simulink model "EPA_Jumpe_v1"  (R2018a)
settings: Solver=FixedStepDiscrete  StartTime=0.0  StopTime=inf  FixedStep=0.001  RelTol=1e-3  EnableMultiTasking=on
model workspace (MAT data in the model file):
  k_p_pam = Simulink.Parameter
  k_p_pam.DataType = 'auto'
  k_p_pam.Dimensions = [0 0]
values from neighbouring files (symbols this model uses):
  bits_current = 12    [Init_EPA_Jumper.m]
  bits_GRF = 12    [Init_EPA_Jumper.m]
  bits_Kd = 12    [Init_EPA_Jumper.m]
  bits_Kp = 12    [Init_EPA_Jumper.m]
  bits_position = 16    [Init_EPA_Jumper.m]
  bits_velocity = 12    [Init_EPA_Jumper.m]
  deadzone_in_TIB = 0.45    [Init_EPA_Jumper.m]
  deadzone_out_TIB = 0.48    [Init_EPA_Jumper.m]
  GRF_MAX = 3.3    [Init_EPA_Jumper.m]
  GRF_MIN = 0    [Init_EPA_Jumper.m]
  k_p_TIB = 1    [Init_EPA_Jumper.m]
  KD_MAX = 5.0    (= 5)    [Init_EPA_Jumper.m]
  KD_MIN = 0.0    (= 0)    [Init_EPA_Jumper.m]
  KP_MAX = 500.0    (= 500)    [Init_EPA_Jumper.m]
  KP_MIN = 0.0    (= 0)    [Init_EPA_Jumper.m]
  P_MAX = 95.5    [Init_EPA_Jumper.m]
  P_MIN = -95.5    [Init_EPA_Jumper.m]
  PressureFilter_CutOffFreq = 50    [Init_EPA_Jumper.m]
  PressureFilter_Gain = 1    [Init_EPA_Jumper.m]
  ReadingVoltage = 5    [Init_EPA_Jumper.m]
  T_MAX = 18.0    (= 18)    [Init_EPA_Jumper.m]
  T_MIN = -18.0    (= -18)    [Init_EPA_Jumper.m]
  V_MAX = 45.0    (= 45)    [Init_EPA_Jumper.m]
  V_MIN = -45.0    (= -45)    [Init_EPA_Jumper.m]
  voltageBias_GAS = -2.3721    [Init_EPA_Jumper.m]
  voltageBias_GL = -2.2892    [Init_EPA_Jumper.m]
  voltageBias_HAM = -2.3721    [Init_EPA_Jumper.m]
  voltageBias_IL = -2.3721    [Init_EPA_Jumper.m]
  voltageBias_POP = -2.3721    [Init_EPA_Jumper.m]
  voltageBias_RF = -2.3721    [Init_EPA_Jumper.m]
  voltageBias_SOL = -2.3721    [Init_EPA_Jumper.m]
  voltageBias_TIB = -2.3721    [Init_EPA_Jumper.m]
  voltageBias_VAS = -2.3721    [Init_EPA_Jumper.m]
  voltageMultiplier_GAS = 2.4915    [Init_EPA_Jumper.m]
  voltageMultiplier_GL = 2.5259    [Init_EPA_Jumper.m]
  voltageMultiplier_HAM = 2.4915    [Init_EPA_Jumper.m]
  voltageMultiplier_IL = 2.4915    [Init_EPA_Jumper.m]
  voltageMultiplier_POP = 2.4915    [Init_EPA_Jumper.m]
  voltageMultiplier_RF = 2.4915    [Init_EPA_Jumper.m]
  voltageMultiplier_SOL = 2.4915    [Init_EPA_Jumper.m]
  voltageMultiplier_TIB = 2.4915    [Init_EPA_Jumper.m]
  voltageMultiplier_VAS = 2.4915    [Init_EPA_Jumper.m]
  VoltageResolution = 1024.0    (= 1024)    [Init_EPA_Jumper.m]
libraries: xpcethercatlib x75, simulink x10, peGeneralControl x9, slrtlib x9
(part 1 of 3)
settings Model: xpc_rtwmakecfg_data=_xpcethercatlib_  SimulationMode=external  Creator=marcm  LastModifiedBy=marcm
settings SolverCC: ConcurrentTasks=on  AutoInsertRateTranBlk=on
settings DataIOCC: SaveFormat=StructureWithTime
settings OptimizationCC: BlockReduction=off  OptimizeBlockIOStorage=off  BufferReuse=off  GlobalBufferReuse=off  ExpressionFolding=off  LocalBlockOutputs=off  OptimizeDataStoreBuffers=off  BusAssignmentInplaceUpdate=off
settings HardwareCC: ProdBitPerPointer=32  ProdBitPerSizeT=32  ProdBitPerPtrDiffT=32  ProdLargestAtomicFloat=None  ProdWordSize=32  ProdLongLongMode=on  ProdHWDeviceType=Generic->32-bit x86 compatible
settings RTWCC: SystemTargetFile=slrt.tlc  TemplateMakefile=slrt_default_tmf  Description=Simulink Real-Time  CodeExecutionProfiling=on  RTWCompilerOptimization=on
settings CodeAppCC: StateflowObjectComments=on
settings SimulinkRealTimeCC: SupportVariableSizeSignals=on  xPCConcurrentTasks=on

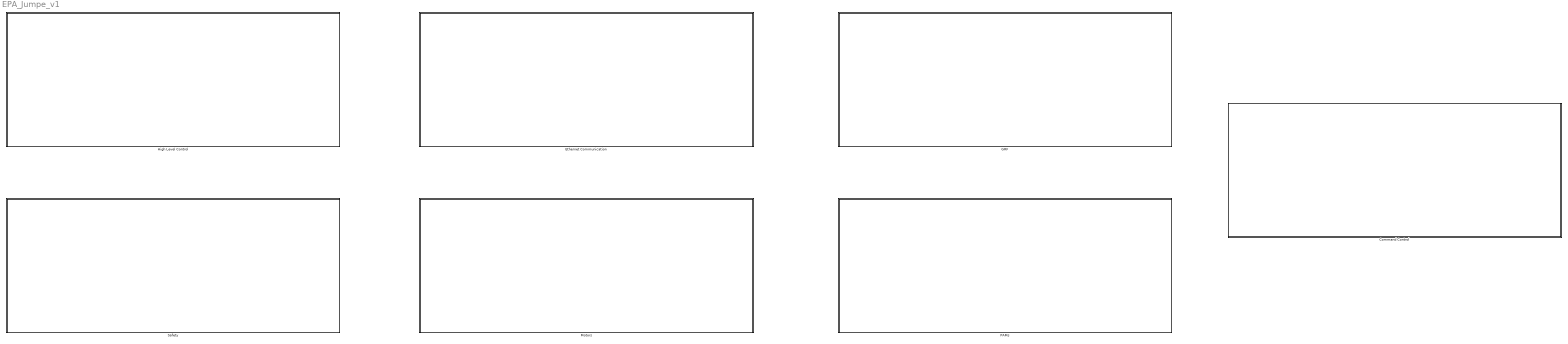
== system EPA_Jumpe_v1 ==
  Command Control : Subsystem
  Ethernet Communication : Subsystem
  GRF : Subsystem
  High Level Control : Subsystem
  Motors : Subsystem
  PAMs : Subsystem
  "Safety " : Subsystem

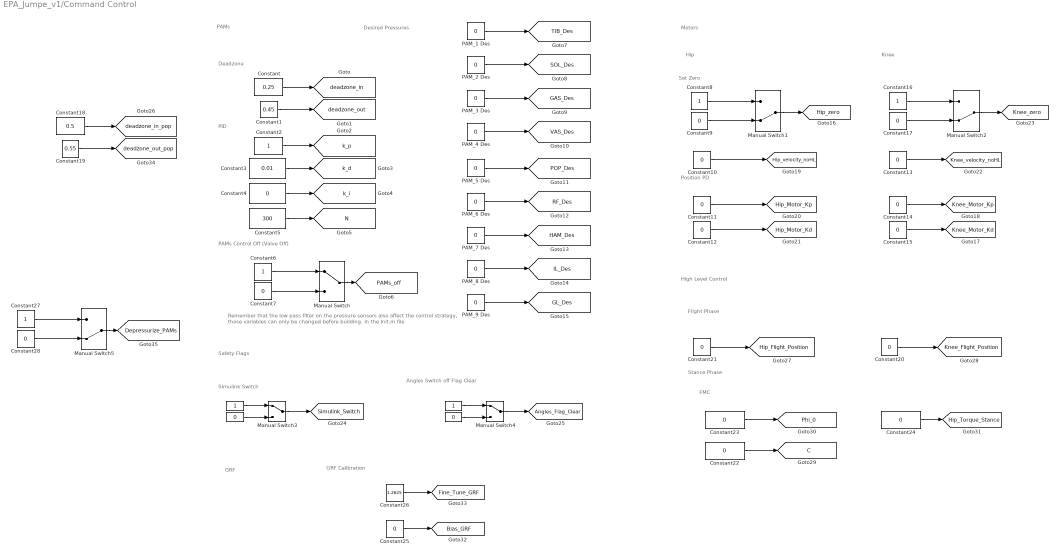
== system EPA_Jumpe_v1/Command Control ==
  note: PID
  note: PAMs
  note: Deadzone
  note: PAMs Control Off (Valve Off)
  note: Desired Pressures
  note: Motors
  note: Remember that the low pass filter on the pressure sensors also affect the control strategy, those variables can only be changed before building. In the Init.m file
  note: Hip
  note: Knee
  note: Safety Flags
  note: Simulink Switch
  note: Angles Switch off Flag Clear
  note: GRF
  note: High Level Control
  note: Flight Phase
  note: Stance Phase
  note: FMC
  note: Position PD
  note: Set Zero
  note: GRF Calibration
  " " : Constant
  "   " : Constant  Value=0
  "    " : Constant  Value=0
  "               " : Constant
  Constant : Constant  Value=0.25
  Constant1 : Constant  Value=0.45
  Constant{4,7,9..15,17,20..25,28} (17 alike) : Constant  Value=0
  Constant{2,6,8,16,27} (5 alike) : Constant
  Constant18 : Constant  Value=0.5
  Constant19 : Constant  Value=0.55
  Constant26 : Constant  Value=1.2625
  Constant3 : Constant  Value=0.01
  Constant5 : Constant  Value=300
  Manual Switch : ManualSwitch
  Manual Switch1 : ManualSwitch  CurrentSetting=0
  Manual Switch2 : ManualSwitch  CurrentSetting=0
  Manual Switch3 : ManualSwitch
  Manual Switch4 : ManualSwitch
  Manual Switch5 : ManualSwitch  CurrentSetting=0
  PAM_1 Des : Constant  Value=0
  PAM_2 Des : Constant  Value=0
  PAM_3 Des : Constant  Value=0
  PAM_4 Des : Constant  Value=0
  PAM_5 Des : Constant  Value=0
  PAM_6 Des : Constant  Value=0
  PAM_7 Des : Constant  Value=0
  PAM_8 Des : Constant  Value=0
  PAM_9 Des : Constant  Value=0
  tag scope: Angles_Flag_Clear=global, Bias_GRF=global, C=global, Depressurize_PAMs=global, Fine_Tune_GRF=global, GAS_Des=global, GL_Des=global, HAM_Des=global, Hip_Flight_Position=global, Hip_Motor_Kd=global, Hip_Motor_Kp=global, Hip_Torque_Stance=global, Hip_velocity_noHL=global, Hip_zero=global, IL_Des=global, Knee_Flight_Position=global, Knee_Motor_Kd=global, Knee_Motor_Kp=global, Knee_velocity_noHL=global, Knee_zero=global, N=global, PAMs_off=global, POP_Des=global, Phi_0=global, RF_Des=global, SOL_Des=global, Simulink_Switch=global, TIB_Des=global, VAS_Des=global, deadzone_in=global, deadzone_in_pop=global, deadzone_out=global, deadzone_out_pop=global, k_d=global, k_i=global, k_p=global
  wires:
  Constant5/1 -> [N]
  Constant4/1 -> [k_i]
  Constant6/1 -> Manual Switch/1
  Manual Switch/1 -> [PAMs_off]
  Constant1/1 -> [deadzone_out]
  Constant7/1 -> Manual Switch/2
  Constant2/1 -> [k_p]
  Constant/1 -> [deadzone_in]
  Constant3/1 -> [k_d]
  PAM_1 Des/1 -> [TIB_Des]
  PAM_2 Des/1 -> [SOL_Des]
  PAM_3 Des/1 -> [GAS_Des]
  PAM_4 Des/1 -> [VAS_Des]
  PAM_5 Des/1 -> [POP_Des]
  PAM_6 Des/1 -> [RF_Des]
  PAM_7 Des/1 -> [HAM_Des]
  PAM_8 Des/1 -> [IL_Des]
  PAM_9 Des/1 -> [GL_Des]
  Constant8/1 -> Manual Switch1/1
  Constant9/1 -> Manual Switch1/2
  Manual Switch1/1 -> [Hip_zero]
  Constant10/1 -> [Hip_velocity_noHL]
  Constant11/1 -> [Hip_Motor_Kp]
  Constant12/1 -> [Hip_Motor_Kd]
  Constant13/1 -> [Knee_velocity_noHL]
  Constant14/1 -> [Knee_Motor_Kp]
  Constant15/1 -> [Knee_Motor_Kd]
  Manual Switch2/1 -> [Knee_zero]
  Constant17/1 -> Manual Switch2/2
  Constant16/1 -> Manual Switch2/1
  " "/1 -> Manual Switch3/1
  "    "/1 -> Manual Switch3/2
  Manual Switch3/1 -> [Simulink_Switch]
  Manual Switch4/1 -> [Angles_Flag_Clear]
  "               "/1 -> Manual Switch4/1
  "   "/1 -> Manual Switch4/2
  Constant21/1 -> [Hip_Flight_Position]
  Constant20/1 -> [Knee_Flight_Position]
  Constant23/1 -> [Phi_0]
  Constant22/1 -> [C]
  Constant24/1 -> [Hip_Torque_Stance]
  Constant25/1 -> [Bias_GRF]
  Constant26/1 -> [Fine_Tune_GRF]
  Constant18/1 -> [deadzone_in_pop]
  Constant19/1 -> [deadzone_out_pop]
  Constant27/1 -> Manual Switch5/1
  Constant28/1 -> Manual Switch5/2
  Manual Switch5/1 -> [Depressurize_PAMs]

== system EPA_Jumpe_v1/Ethernet Communication ==
  "EtherCAT Get Notifications " : xpcethercatlib/EtherCAT Get Notifications   device_id=0  sample_time=.001
      settings: SourceProductName=Simulink Real-Time  SourceProductBaseCode=XP
  "EtherCAT Init " : xpcethercatlib/EtherCAT Init   Priority=0  config_file=C:\Users\marcm\PhD\EPA-Jumper\RealTime Code\EPA Jumper v1\EPA_Jumper_xml.xml  device_id=0  pci_bus=3  pci_slot=0  pci_function=0  dctuning=0  enaDebug=off  enaDC=on  errLink=off  masterDbg=off  stateChgDbg=off  baseClock=off  masterCfg=off  logFile='c:\dbglog.txt'  sample_time=0.001000  DCMode=0
      settings: SourceProductName=Simulink Real-Time  SourceProductBaseCode=XP
  Inputs : Subsystem
  Outputs : Subsystem
  Terminator : Terminator
  Terminator1 : Terminator
  wires:
  "EtherCAT Get Notifications "/1 -> Terminator1/1
  "EtherCAT Init "/1 -> Terminator/1

== system EPA_Jumpe_v1/GRF ==
  note: GRF Meassures
  2D-Vector : Subsystem
  GRFx : Subsystem
  GRFy : Subsystem
  GRFz : Subsystem

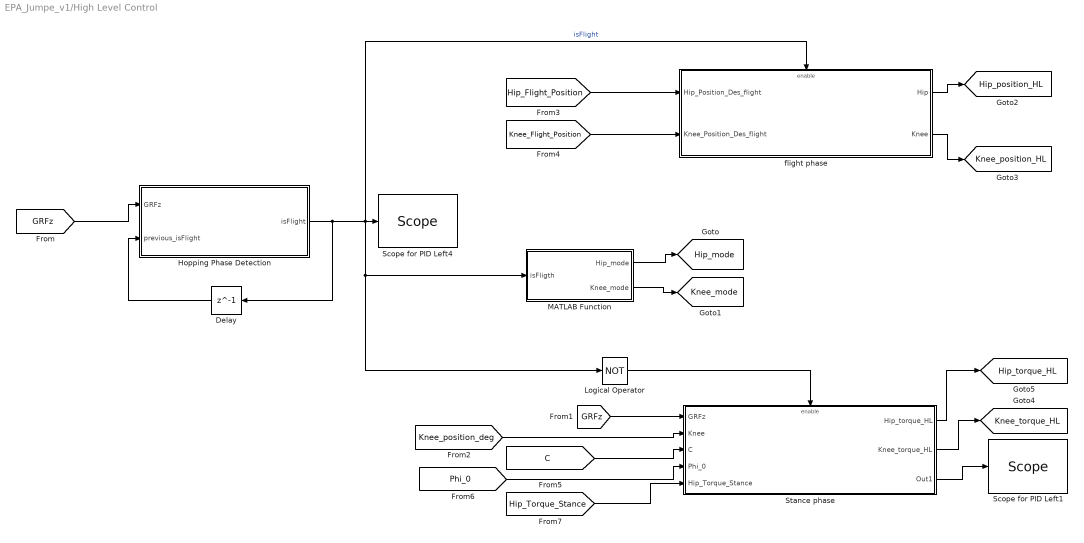
== system EPA_Jumpe_v1/High Level Control ==
  Delay : Delay  DelayLength=1
  Hopping Phase Detection : MATLAB Function  TreatAsAtomicUnit=on
  Logical Operator : Logic  Operator=NOT  AllPortsSameDT=off  OutDataTypeStr=boolean
  MATLAB Function : MATLAB Function  TreatAsAtomicUnit=on
  Scope for PID Left1 : slrtlib/Displays and Logging/Scope   scopeno=7  scopetype=Target  autostart=on  viewmode=Numerical  formatstr='%15.6f'  grid=on  ylimits=[-60, 60]  nosamples=1000  noprepostsamples=0  interleave=1  triggermode=FreeRun  triggersignal=1  trigsignalfromport=off  triggerlevel=0.0  triggerslope=Either  triggerscope=1  triggersample=0  filename=data.dat  mode=Lazy  writesize=512  autorestart=off  dynamicfilemode=off  maxwritefilesize=512*1024^2
  Scope for PID Left4 : slrtlib/Displays and Logging/Scope   scopeno=6  scopetype=Target  autostart=on  viewmode=Graphical sliding  formatstr='%15.6f'  grid=on  ylimits=[0, 0]  nosamples=1000  noprepostsamples=0  interleave=1  triggermode=FreeRun  triggersignal=1  trigsignalfromport=off  triggerlevel=0.0  triggerslope=Either  triggerscope=1  triggersample=0  filename=data.dat  mode=Lazy  writesize=512  autorestart=off  dynamicfilemode=off  maxwritefilesize=512*1024^2
  Stance phase : Subsystem
  flight phase : Subsystem
  tag scope: Hip_mode=global, Hip_position_HL=global, Hip_torque_HL=global, Knee_mode=global, Knee_position_HL=global, Knee_torque_HL=global
  wires:
  Hopping Phase Detection/1(isFlight) -> Delay/1, flight phase/Enable, Scope for PID Left4/1, MATLAB Function/1(isFligth), Logical Operator/1  "isFlight"
  [GRFz] -> Hopping Phase Detection/1(GRFz)
  [Hip_Flight_Position] -> flight phase/1(Hip_Position_Des_flight)
  [Knee_Flight_Position] -> flight phase/2(Knee_Position_Des_flight)
  Logical Operator/1 -> Stance phase/Enable
  MATLAB Function/1(Hip_mode) -> [Hip_mode]
  MATLAB Function/2(Knee_mode) -> [Knee_mode]
  flight phase/1(Hip) -> [Hip_position_HL]
  flight phase/2(Knee) -> [Knee_position_HL]
  [GRFz] -> Stance phase/1("GRFz ")
  [Knee_position_deg] -> Stance phase/2(Knee)
  Stance phase/2(Knee_torque_HL) -> [Knee_torque_HL]
  Stance phase/3(Out1) -> Scope for PID Left1/1
  Stance phase/1(Hip_torque_HL) -> [Hip_torque_HL]
  [C] -> Stance phase/3(C)
  [Phi_0] -> Stance phase/4(Phi_0)
  [Hip_Torque_Stance] -> Stance phase/5(Hip_Torque_Stance)
  Delay/1 -> Hopping Phase Detection/2(previous_isFlight)

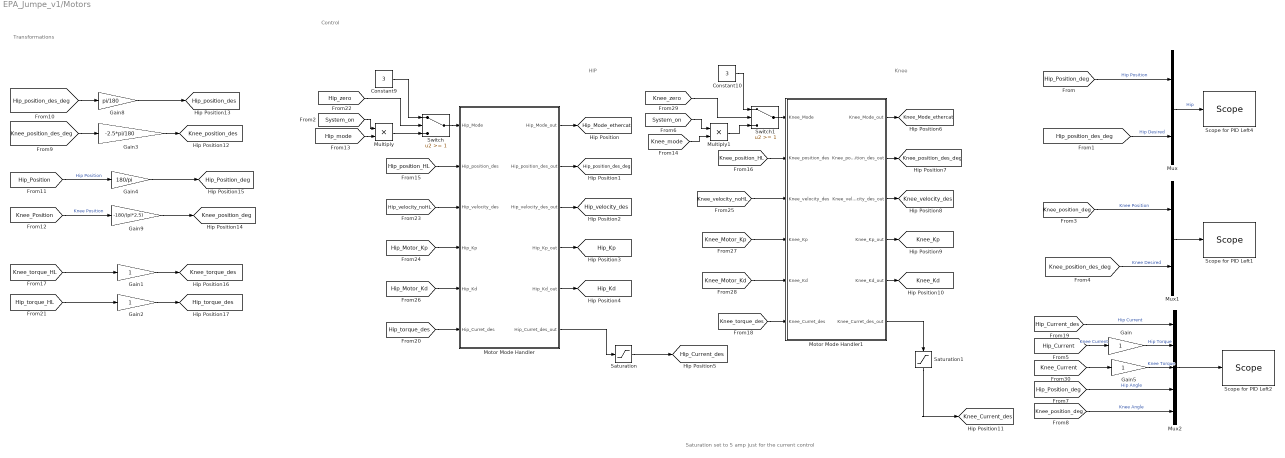
== system EPA_Jumpe_v1/Motors ==
  note: Saturation set to 5 amp just for the current control
  note: HIP
  note: Knee
  note: Control
  note: Transformations
  Constant10 : Constant  Value=3
  Constant9 : Constant  Value=3
  Gain{,1..2,5} (4 alike) : Gain
  Gain3 : Gain  Gain=-2.5*pi/180
  Gain4 : Gain  Gain=180/pi
  Gain8 : Gain  Gain=pi/180
  Gain9 : Gain  Gain=-180/(pi*2.5)
  Motor Mode Handler : MATLAB Function  TreatAsAtomicUnit=on
  Motor Mode Handler1 : MATLAB Function  TreatAsAtomicUnit=on
  Multiply : Product
  Multiply1 : Product
  Mux : Mux  Inputs=2
  Mux1 : Mux  Inputs=2
  Mux2 : Mux  Inputs=5
  Saturation : Saturate  UpperLimit=5  LowerLimit=-5
  Saturation1 : Saturate  UpperLimit=5  LowerLimit=-5
  Scope for PID Left1 : slrtlib/Displays and Logging/Scope   scopeno=4  scopetype=Target  autostart=on  viewmode=Graphical sliding  formatstr='%15.6f'  grid=on  ylimits=[0, 120]  nosamples=1000  noprepostsamples=0  interleave=1  triggermode=FreeRun  triggersignal=1  trigsignalfromport=off  triggerlevel=0.0  triggerslope=Either  triggerscope=1  triggersample=0  filename=data.dat  mode=Lazy  writesize=512  autorestart=off  dynamicfilemode=off  maxwritefilesize=512*1024^2
  Scope for PID Left2 : slrtlib/Displays and Logging/Scope   scopeno=5  scopetype=Target  autostart=on  viewmode=Numerical  formatstr='%15.6f'  grid=on  ylimits=[0, 0]  nosamples=1000  noprepostsamples=0  interleave=1  triggermode=FreeRun  triggersignal=1  trigsignalfromport=off  triggerlevel=0.0  triggerslope=Either  triggerscope=1  triggersample=0  filename=data.dat  mode=Lazy  writesize=512  autorestart=off  dynamicfilemode=off  maxwritefilesize=512*1024^2
  Scope for PID Left4 : slrtlib/Displays and Logging/Scope   scopeno=3  scopetype=Target  autostart=on  viewmode=Graphical sliding  formatstr='%15.6f'  grid=on  ylimits=[-60, 60]  nosamples=1000  noprepostsamples=0  interleave=1  triggermode=FreeRun  triggersignal=1  trigsignalfromport=off  triggerlevel=0.0  triggerslope=Either  triggerscope=1  triggersample=0  filename=data.dat  mode=Lazy  writesize=512  autorestart=off  dynamicfilemode=off  maxwritefilesize=512*1024^2
  Switch : Switch  Threshold=1
  Switch1 : Switch  Threshold=1
  tag scope: Hip_Current_des=global, Hip_Kd=global, Hip_Kp=global, Hip_Mode_ethercat=global, Hip_Position_deg=global, Hip_position_des=global, Hip_position_des_deg=global, Hip_torque_des=global, Hip_velocity_des=global, Knee_Current_des=global, Knee_Kd=global, Knee_Kp=global, Knee_Mode_ethercat=global, Knee_position_deg=global, Knee_position_des=global, Knee_position_des_deg=global, Knee_torque_des=global, Knee_velocity_des=global
  wires:
  Motor Mode Handler/3(Hip_velocity_des_out) -> [Hip_velocity_des]
  Motor Mode Handler/4(Hip_Kp_out) -> [Hip_Kp]
  Motor Mode Handler/5(Hip_Kd_out) -> [Hip_Kd]
  Motor Mode Handler/6(Hip_Curret_des_out) -> Saturation/1
  Motor Mode Handler/2(Hip_position_des_out) -> [Hip_position_des_deg]
  [Hip_position_des_deg] -> Mux/2  "Hip Desired"
  [Hip_Position_deg] -> Mux/1  "Hip Position"
  Mux/1 -> Scope for PID Left4/1  "Hip"
  Mux1/1 -> Scope for PID Left1/1
  [Knee_position_des_deg] -> Mux1/2  "Knee Desired"
  [Hip_Current] -> Gain/1  "Knee Current"
  [Hip_Current_des] -> Mux2/1  "Hip Current"
  Mux2/1 -> Scope for PID Left2/1
  Multiply/1 -> Switch/3
  [System_on] -> Multiply/1
  Motor Mode Handler/1(Hip_Mode_out) -> [Hip_Mode_ethercat]
  [Hip_position_HL] -> Motor Mode Handler/2(Hip_position_des)
  [Hip_velocity_noHL] -> Motor Mode Handler/3(Hip_velocity_des)
  [Hip_Motor_Kp] -> Motor Mode Handler/4(Hip_Kp)
  [Hip_Motor_Kd] -> Motor Mode Handler/5(Hip_Kd)
  [Hip_torque_des] -> Motor Mode Handler/6(Hip_Curret_des)
  [Knee_position_HL] -> Motor Mode Handler1/2(Knee_position_des)
  [System_on] -> Multiply1/1
  Motor Mode Handler1/5(Knee_Kd_out) -> [Knee_Kd]
  Motor Mode Handler1/1(Knee_Mode_out) -> [Knee_Mode_ethercat]
  Motor Mode Handler1/2(Knee_position_des_out) -> [Knee_position_des_deg]
  Motor Mode Handler1/3(Knee_velocity_des_out) -> [Knee_velocity_des]
  Motor Mode Handler1/4(Knee_Kp_out) -> [Knee_Kp]
  Motor Mode Handler1/6(Knee_Curret_des_out) -> Saturation1/1
  [Knee_position_deg] -> Mux1/1  "Knee Position"
  [Hip_position_des_deg] -> Gain8/1
  [Knee_position_des_deg] -> Gain3/1
  [Hip_Position] -> Gain4/1  "Hip Position"
  [Knee_Position] -> Gain9/1  "Knee Position"
  Gain3/1 -> [Knee_position_des]
  Gain8/1 -> [Hip_position_des]
  Gain9/1 -> [Knee_position_deg]
  Gain4/1 -> [Hip_Position_deg]
  [Knee_torque_HL] -> Gain1/1
  Gain1/1 -> [Knee_torque_des]
  [Hip_mode] -> Multiply/2
  Constant9/1 -> Switch/1
  [Knee_mode] -> Multiply1/2
  Constant10/1 -> Switch1/1
  Switch/1 -> Motor Mode Handler/1(Hip_Mode)
  Switch1/1 -> Motor Mode Handler1/1(Knee_Mode)
  [Knee_torque_des] -> Motor Mode Handler1/6(Knee_Curret_des)
  Saturation/1 -> [Hip_Current_des]
  Saturation1/1 -> [Knee_Current_des]
  [Hip_torque_HL] -> Gain2/1
  Gain2/1 -> [Hip_torque_des]
  [Hip_zero] -> Switch/2
  [Knee_velocity_noHL] -> Motor Mode Handler1/3(Knee_velocity_des)
  [Knee_Motor_Kp] -> Motor Mode Handler1/4(Knee_Kp)
  [Knee_Motor_Kd] -> Motor Mode Handler1/5(Knee_Kd)
  Multiply1/1 -> Switch1/3
  [Knee_zero] -> Switch1/2
  [Knee_position_deg] -> Mux2/5  "Knee Angle"
  [Hip_Position_deg] -> Mux2/4  "Hip Angle"
  [Knee_Current] -> Gain5/1
  Gain/1 -> Mux2/2  "Hip Torque"
  Gain5/1 -> Mux2/3  "Knee Torque"

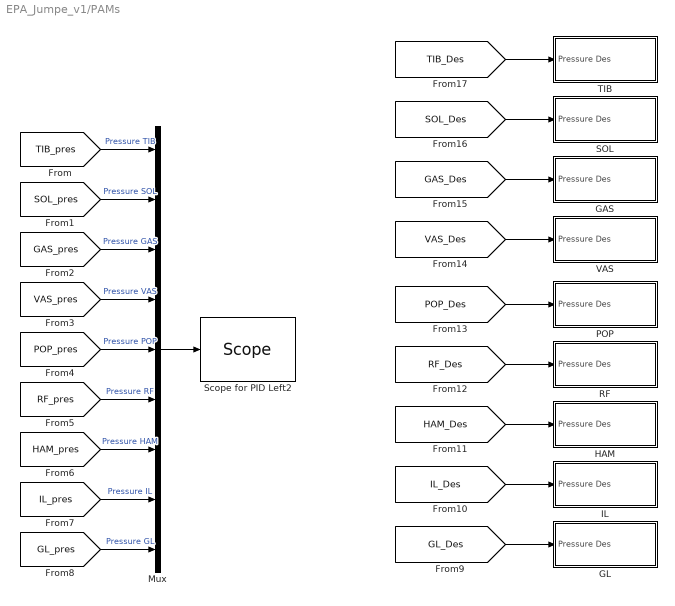
== system EPA_Jumpe_v1/PAMs ==
  GAS : Subsystem
  GL : Subsystem
  HAM : Subsystem
  IL : Subsystem
  Mux : Mux  Inputs=9
  POP : Subsystem
  RF : Subsystem
  SOL : Subsystem
  Scope for PID Left2 : slrtlib/Displays and Logging/Scope   scopeno=8  scopetype=Target  autostart=on  viewmode=Numerical  formatstr='%15.6f'  grid=on  ylimits=[0, 0]  nosamples=1000  noprepostsamples=0  interleave=1  triggermode=FreeRun  triggersignal=1  trigsignalfromport=off  triggerlevel=0.0  triggerslope=Either  triggerscope=1  triggersample=0  filename=data.dat  mode=Lazy  writesize=512  autorestart=off  dynamicfilemode=off  maxwritefilesize=512*1024^2
  TIB : Subsystem
  VAS : Subsystem
  wires:
  Mux/1 -> Scope for PID Left2/1
  [TIB_pres] -> Mux/1  "Pressure TIB"
  [SOL_pres] -> Mux/2  "Pressure SOL"
  [GAS_pres] -> Mux/3  "Pressure GAS"
  [VAS_pres] -> Mux/4  "Pressure VAS"
  [POP_pres] -> Mux/5  "Pressure POP"
  [RF_pres] -> Mux/6  "Pressure RF"
  [HAM_pres] -> Mux/7  "Pressure HAM"
  [IL_pres] -> Mux/8  "Pressure IL"
  [GL_pres] -> Mux/9  "Pressure GL"
  [TIB_Des] -> TIB/1(Pressure Des)
  [SOL_Des] -> SOL/1(Pressure Des)
  [GAS_Des] -> GAS/1(Pressure Des)
  [VAS_Des] -> VAS/1(Pressure Des)
  [POP_Des] -> POP/1(Pressure Des)
  [RF_Des] -> RF/1(Pressure Des)
  [HAM_Des] -> HAM/1(Pressure Des)
  [IL_Des] -> IL/1(Pressure Des)
  [GL_Des] -> GL/1(Pressure Des)

== system EPA_Jumpe_v1/Safety  ==
  AND1 : Logic  IconShape=distinctive  AllPortsSameDT=off  OutDataTypeStr=boolean
  Delay : Delay  DelayLength=1  InitialCondition=0  ExternalReset=Either
      settings: InputPortMap=u0,r5
  MATLAB Function : MATLAB Function  TreatAsAtomicUnit=on
  Mux : Mux  Inputs=6
  Scope for PID Left4 : slrtlib/Displays and Logging/Scope   scopeno=2  scopetype=Target  autostart=on  viewmode=Numerical  formatstr='%15.6f'  grid=on  ylimits=[0, 0]  nosamples=1000  noprepostsamples=0  interleave=1  triggermode=FreeRun  triggersignal=1  trigsignalfromport=off  triggerlevel=0.0  triggerslope=Either  triggerscope=1  triggersample=0  filename=data.dat  mode=Lazy  writesize=512  autorestart=off  dynamicfilemode=off  maxwritefilesize=512*1024^2
  System On : Subsystem
  tag scope: System_on=global
  wires:
  System On/1(System On) -> Mux/1, AND1/1  "System On"
  [Simulink_Switch] -> Mux/2, System On/1("Simulink Switch ")  "Simulink Switch"
  Mux/1 -> Scope for PID Left4/1
  System On/2(Emergency) -> Mux/3  "Emergency Switch"
  [Hip_Position_deg] -> MATLAB Function/1(Hip_Position)
  MATLAB Function/3(Motors_safe) -> AND1/2, Mux/4  "Motors_safe"
  MATLAB Function/1(Hip_motor_safe) -> Mux/5  "Hip_motor_safe"
  MATLAB Function/2(Knee_motor_safe) -> Mux/6  "Knee_motor_safe"
  AND1/1 -> [System_on]
  MATLAB Function/4(flag) -> Delay/1
  Delay/1 -> MATLAB Function/3(flag_1)
  [Angles_Flag_Clear] -> Delay/2
  [Knee_position_deg] -> MATLAB Function/2(Knee_Position)

== system EPA_Jumpe_v1/Ethernet Communication/Inputs ==
  GRF Slave : Subsystem
  Motor Slave : Subsystem
  PAMs Slave : Subsystem

== system EPA_Jumpe_v1/Ethernet Communication/Outputs ==
  GRF Slave : Subsystem
  Motor Slave : Subsystem
  PAMs Slave : Subsystem

== system EPA_Jumpe_v1/GRF/2D-Vector ==
  Asin : Trigonometry  Operator=asin
  Divide : Product  Inputs=*/
  Sqrt : Sqrt  SaturateOnIntegerOverflow=on
  Square : Math  Operator=square  SaturateOnIntegerOverflow=on
  Square1 : Math  Operator=square  SaturateOnIntegerOverflow=on
  Sum : Sum  Inputs=+|+
  tag scope: GRF_VectAng=global, GRF_VectMag=global
  wires:
  [GRFy] -> Square/1
  [GRFz] -> Square1/1
  Square/1 -> Sum/1
  Square1/1 -> Divide/1, Sum/2
  Sum/1 -> Sqrt/1
  Sqrt/1 -> Divide/2, [GRF_VectMag]  "GRF Vector"
  Divide/1 -> Asin/1
  Asin/1 -> [GRF_VectAng]  "GRF Angle"

== system EPA_Jumpe_v1/GRF/GRFx ==
  note: GRF Low Pass Filter
  Constant17 : Constant  Value=0
  Constant18 : Constant
  Filter : DiscreteFilter  Numerator="[0.0036    0.0072    0.0036]"  Denominator="[1.0000   -1.8227    0.8372]"  ExternalReset=Either
      settings: InputPortMap=u0,r7
  Gain27 : Gain  Gain=100
  Sum3 : Sum  Inputs=|+-
  tag scope: GRFx=global
  wires:
  Gain27/1 -> Sum3/1
  Sum3/1 -> Filter/1
  Filter/1 -> [GRFx]  "GRF z"
  Constant17/1 -> Sum3/2
  Constant18/1 -> Filter/2
  [GRFx_Volts] -> Gain27/1

== system EPA_Jumpe_v1/GRF/GRFy ==
  note: GRF Low Pass Filter
  Constant17 : Constant  Value=0
  Constant18 : Constant
  Filter : DiscreteFilter  Numerator="[0.0036    0.0072    0.0036]"  Denominator="[1.0000   -1.8227    0.8372]"  ExternalReset=Either
      settings: InputPortMap=u0,r7
  Gain27 : Gain  Gain=200
  Scope for PID Left4 : slrtlib/Displays and Logging/Scope   scopeno=9  scopetype=Target  autostart=on  viewmode=Graphical sliding  formatstr='%15.6f'  grid=on  ylimits=[0, 0]  nosamples=1000  noprepostsamples=0  interleave=1  triggermode=FreeRun  triggersignal=1  trigsignalfromport=off  triggerlevel=0.0  triggerslope=Either  triggerscope=1  triggersample=0  filename=data.dat  mode=Lazy  writesize=512  autorestart=off  dynamicfilemode=off  maxwritefilesize=512*1024^2
  Sum3 : Sum  Inputs=|+-
  tag scope: GRFy=global
  wires:
  Gain27/1 -> Sum3/1
  Sum3/1 -> Filter/1
  Filter/1 -> Scope for PID Left4/1, [GRFy]  "GRF y"
  Constant17/1 -> Sum3/2
  Constant18/1 -> Filter/2
  [GRFy_Volts] -> Gain27/1

== system EPA_Jumpe_v1/GRF/GRFz ==
  note: GRF Low Pass Filter
  Constant18 : Constant
  Filter : DiscreteFilter  Numerator="[0.0036    0.0072    0.0036]"  Denominator="[1.0000   -1.8227    0.8372]"  ExternalReset=Either
      settings: InputPortMap=u0,r7
  Gain27 : Gain  Gain=300
  Multiply : Product
  Scope for PID Left4 : slrtlib/Displays and Logging/Scope   scopeno=1  scopetype=Target  autostart=on  viewmode=Graphical sliding  formatstr='%15.6f'  grid=on  ylimits=[0, 0]  nosamples=1000  noprepostsamples=0  interleave=1  triggermode=FreeRun  triggersignal=1  trigsignalfromport=off  triggerlevel=0.0  triggerslope=Either  triggerscope=1  triggersample=0  filename=data.dat  mode=Lazy  writesize=512  autorestart=off  dynamicfilemode=off  maxwritefilesize=512*1024^2
  Sum3 : Sum  Inputs=|+-
  tag scope: GRFz=global
  wires:
  Constant18/1 -> Filter/2
  [Bias_GRF] -> Sum3/2
  Sum3/1 -> Filter/1
  [GRFz_Volts] -> Gain27/1
  Filter/1 -> Scope for PID Left4/1, [GRFz]  "GRF z"
  Gain27/1 -> Multiply/1
  Multiply/1 -> Sum3/1
  [Fine_Tune_GRF] -> Multiply/2

== system EPA_Jumpe_v1/High Level Control/Stance phase ==
  "GRFz " : Inport
  Knee : Inport  Port=2
  C : Inport  Port=3
  Phi_0 : Inport  Port=4
  Hip_Torque_Stance : Inport  Port=5
  Enable : EnablePort  StatesWhenEnabling=reset
  FMCK (Static) : Subsystem
  Mux : Mux  Inputs=2
  Hip_torque_HL : Outport
  Knee_torque_HL : Outport  Port=2
  Out1 : Outport  Port=3
  wires:
  "GRFz "/1 -> FMCK (Static)/1(GRF_Z)
  Knee/1 -> FMCK (Static)/2(angKne)
  FMCK (Static)/2(Phi0) -> Mux/1
  Mux/1 -> Out1/1
  FMCK (Static)/3(C) -> Mux/2
  FMCK (Static)/1(torMotKne) -> Knee_torque_HL/1
  Hip_Torque_Stance/1 -> Hip_torque_HL/1
  C/1 -> FMCK (Static)/3(C_)
  Phi_0/1 -> FMCK (Static)/4(Phi_0)

== system EPA_Jumpe_v1/High Level Control/flight phase ==
  Hip_Position_Des_flight : Inport
  Knee_Position_Des_flight : Inport  Port=2
  Enable : EnablePort  StatesWhenEnabling=reset
  Hip : Outport
  Knee : Outport  Port=2
  wires:
  Hip_Position_Des_flight/1 -> Hip/1
  Knee_Position_Des_flight/1 -> Knee/1

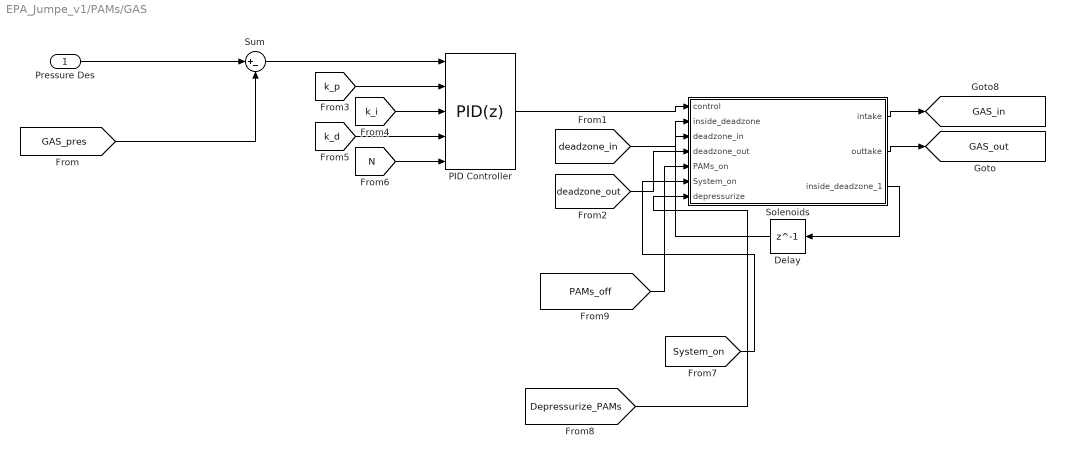
== system EPA_Jumpe_v1/PAMs/GAS ==
  Pressure Des : Inport
  Delay : Delay  DelayLength=1
  PID Controller : simulink/Continuous/PID Controller  Controller=PID  TimeDomain=Discrete-time  SampleTime=-1  IntegratorMethod=Forward Euler  FilterMethod=Forward Euler  Form=Ideal  UseFilter=on  ControllerParametersSource=external  P=k_p_pam  I=0  D=0.45*0.15/8  N=100  InitialConditionSource=internal  InitialConditionForIntegrator=0  InitialConditionForFilter=0  ExternalReset=none  LimitOutput=off  UpperSaturationLimit=inf  LowerSaturationLimit=-inf  LinearizeAsGain=on  AntiWindupMode=none  Kb=1  TrackingMode=off  Kt=1  PParamMin=[]  PParamMax=[]  IParamMin=[]  IParamMax=[]  DParamMin=[]  DParamMax=[]  NParamMin=[]  NParamMax=[]  KbParamMin=[]  KbParamMax=[]  KtParamMin=[]  KtParamMax=[]  POutMin=[]  POutMax=[]  IOutMin=[]  IOutMax=[]  DOutMin=[]  DOutMax=[]  NOutMin=[]  NOutMax=[]  KbOutMin=[]  KbOutMax=[]  KtOutMin=[]  KtOutMax=[]  IntegratorOutMin=[]  IntegratorOutMax=[]  FilterOutMin=[]  FilterOutMax=[]  SumOutMin=[]  SumOutMax=[]  SumI1OutMin=[]  SumI1OutMax=[]  SumI2OutMin=[]  SumI2OutMax=[]  SumI3OutMin=[]  SumI3OutMax=[]  SumDOutMin=[]  SumDOutMax=[]  SaturationOutMin=[]  SaturationOutMax=[]  IntegratorContinuousStateAttributes=''  IntegratorStateMustResolveToSignalObject=off  IntegratorRTWStateStorageClass=Auto  FilterContinuousStateAttributes=''  FilterStateMustResolveToSignalObject=off  FilterRTWStateStorageClass=Auto  DifferentiatorICPrevScaledInput=0  DifferentiatorOutMin=[]  DifferentiatorOutMax=[]  FilterDiffOutCoefMin=[]  FilterDiffOutCoefMax=[]  SumDenOutMin=[]  SumDenOutMax=[]  SumNumOutMin=[]  SumNumOutMax=[]  ReciprocalOutMin=[]  ReciprocalOutMax=[]  DivideOutMin=[]  DivideOutMax=[]  TunerSelectOption=Transfer Function Based (PID Tuner App)
  Solenoids : MATLAB Function  TreatAsAtomicUnit=on
  Sum : Sum  Inputs=|+-
  tag scope: GAS_in=global, GAS_out=global
  wires:
  Solenoids/3(inside_deadzone_1) -> Delay/1
  Delay/1 -> Solenoids/2(inside_deadzone)
  Pressure Des/1 -> Sum/1
  [GAS_pres] -> Sum/2
  [deadzone_in] -> Solenoids/3(deadzone_in)
  [deadzone_out] -> Solenoids/4(deadzone_out)
  Solenoids/1(intake) -> [GAS_in]
  Solenoids/2(outtake) -> [GAS_out]
  [k_i] -> PID Controller/3
  [k_d] -> PID Controller/4
  [N] -> PID Controller/5
  Sum/1 -> PID Controller/1
  PID Controller/1 -> Solenoids/1(control)
  [k_p] -> PID Controller/2
  [PAMs_off] -> Solenoids/5(PAMs_on)
  [System_on] -> Solenoids/6(System_on)
  [Depressurize_PAMs] -> Solenoids/7(depressurize)

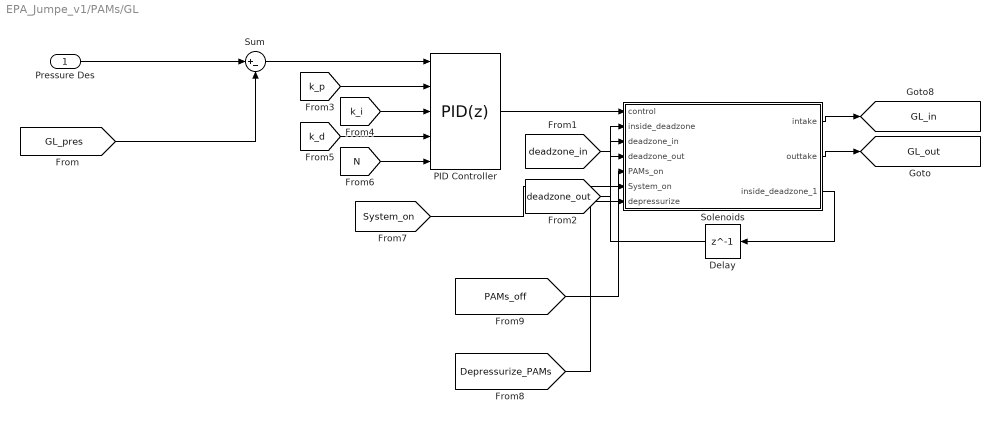
== system EPA_Jumpe_v1/PAMs/GL ==
  Pressure Des : Inport
  Delay : Delay  DelayLength=1
  PID Controller : simulink/Continuous/PID Controller  Controller=PID  TimeDomain=Discrete-time  SampleTime=-1  IntegratorMethod=Forward Euler  FilterMethod=Forward Euler  Form=Ideal  UseFilter=on  ControllerParametersSource=external  P=k_p_pam  I=0  D=0.45*0.15/8  N=100  InitialConditionSource=internal  InitialConditionForIntegrator=0  InitialConditionForFilter=0  ExternalReset=none  LimitOutput=off  UpperSaturationLimit=inf  LowerSaturationLimit=-inf  LinearizeAsGain=on  AntiWindupMode=none  Kb=1  TrackingMode=off  Kt=1  PParamMin=[]  PParamMax=[]  IParamMin=[]  IParamMax=[]  DParamMin=[]  DParamMax=[]  NParamMin=[]  NParamMax=[]  KbParamMin=[]  KbParamMax=[]  KtParamMin=[]  KtParamMax=[]  POutMin=[]  POutMax=[]  IOutMin=[]  IOutMax=[]  DOutMin=[]  DOutMax=[]  NOutMin=[]  NOutMax=[]  KbOutMin=[]  KbOutMax=[]  KtOutMin=[]  KtOutMax=[]  IntegratorOutMin=[]  IntegratorOutMax=[]  FilterOutMin=[]  FilterOutMax=[]  SumOutMin=[]  SumOutMax=[]  SumI1OutMin=[]  SumI1OutMax=[]  SumI2OutMin=[]  SumI2OutMax=[]  SumI3OutMin=[]  SumI3OutMax=[]  SumDOutMin=[]  SumDOutMax=[]  SaturationOutMin=[]  SaturationOutMax=[]  IntegratorContinuousStateAttributes=''  IntegratorStateMustResolveToSignalObject=off  IntegratorRTWStateStorageClass=Auto  FilterContinuousStateAttributes=''  FilterStateMustResolveToSignalObject=off  FilterRTWStateStorageClass=Auto  DifferentiatorICPrevScaledInput=0  DifferentiatorOutMin=[]  DifferentiatorOutMax=[]  FilterDiffOutCoefMin=[]  FilterDiffOutCoefMax=[]  SumDenOutMin=[]  SumDenOutMax=[]  SumNumOutMin=[]  SumNumOutMax=[]  ReciprocalOutMin=[]  ReciprocalOutMax=[]  DivideOutMin=[]  DivideOutMax=[]  TunerSelectOption=Transfer Function Based (PID Tuner App)
  Solenoids : MATLAB Function  TreatAsAtomicUnit=on
  Sum : Sum  Inputs=|+-
  tag scope: GL_in=global, GL_out=global
  wires:
  Solenoids/3(inside_deadzone_1) -> Delay/1
  Delay/1 -> Solenoids/2(inside_deadzone)
  Pressure Des/1 -> Sum/1
  [GL_pres] -> Sum/2
  [deadzone_in] -> Solenoids/3(deadzone_in)
  [deadzone_out] -> Solenoids/4(deadzone_out)
  Solenoids/1(intake) -> [GL_in]
  Solenoids/2(outtake) -> [GL_out]
  [k_i] -> PID Controller/3
  [k_d] -> PID Controller/4
  [N] -> PID Controller/5
  Sum/1 -> PID Controller/1
  PID Controller/1 -> Solenoids/1(control)
  [k_p] -> PID Controller/2
  [PAMs_off] -> Solenoids/5(PAMs_on)
  [System_on] -> Solenoids/6(System_on)
  [Depressurize_PAMs] -> Solenoids/7(depressurize)

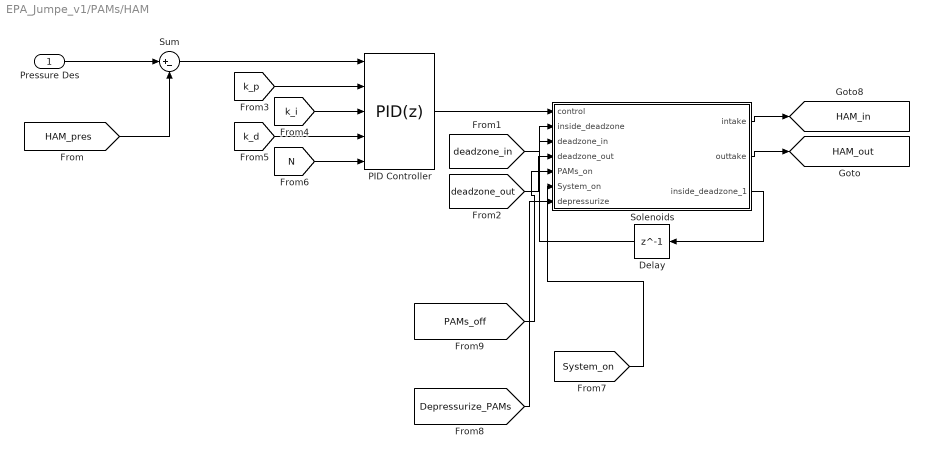
== system EPA_Jumpe_v1/PAMs/HAM ==
  Pressure Des : Inport
  Delay : Delay  DelayLength=1
  PID Controller : simulink/Continuous/PID Controller  Controller=PID  TimeDomain=Discrete-time  SampleTime=-1  IntegratorMethod=Forward Euler  FilterMethod=Forward Euler  Form=Ideal  UseFilter=on  ControllerParametersSource=external  P=k_p_pam  I=0  D=0.45*0.15/8  N=100  InitialConditionSource=internal  InitialConditionForIntegrator=0  InitialConditionForFilter=0  ExternalReset=none  LimitOutput=off  UpperSaturationLimit=inf  LowerSaturationLimit=-inf  LinearizeAsGain=on  AntiWindupMode=none  Kb=1  TrackingMode=off  Kt=1  PParamMin=[]  PParamMax=[]  IParamMin=[]  IParamMax=[]  DParamMin=[]  DParamMax=[]  NParamMin=[]  NParamMax=[]  KbParamMin=[]  KbParamMax=[]  KtParamMin=[]  KtParamMax=[]  POutMin=[]  POutMax=[]  IOutMin=[]  IOutMax=[]  DOutMin=[]  DOutMax=[]  NOutMin=[]  NOutMax=[]  KbOutMin=[]  KbOutMax=[]  KtOutMin=[]  KtOutMax=[]  IntegratorOutMin=[]  IntegratorOutMax=[]  FilterOutMin=[]  FilterOutMax=[]  SumOutMin=[]  SumOutMax=[]  SumI1OutMin=[]  SumI1OutMax=[]  SumI2OutMin=[]  SumI2OutMax=[]  SumI3OutMin=[]  SumI3OutMax=[]  SumDOutMin=[]  SumDOutMax=[]  SaturationOutMin=[]  SaturationOutMax=[]  IntegratorContinuousStateAttributes=''  IntegratorStateMustResolveToSignalObject=off  IntegratorRTWStateStorageClass=Auto  FilterContinuousStateAttributes=''  FilterStateMustResolveToSignalObject=off  FilterRTWStateStorageClass=Auto  DifferentiatorICPrevScaledInput=0  DifferentiatorOutMin=[]  DifferentiatorOutMax=[]  FilterDiffOutCoefMin=[]  FilterDiffOutCoefMax=[]  SumDenOutMin=[]  SumDenOutMax=[]  SumNumOutMin=[]  SumNumOutMax=[]  ReciprocalOutMin=[]  ReciprocalOutMax=[]  DivideOutMin=[]  DivideOutMax=[]  TunerSelectOption=Transfer Function Based (PID Tuner App)
  Solenoids : MATLAB Function  TreatAsAtomicUnit=on
  Sum : Sum  Inputs=|+-
  tag scope: HAM_in=global, HAM_out=global
  wires:
  Solenoids/3(inside_deadzone_1) -> Delay/1
  Delay/1 -> Solenoids/2(inside_deadzone)
  Pressure Des/1 -> Sum/1
  [HAM_pres] -> Sum/2
  [deadzone_in] -> Solenoids/3(deadzone_in)
  [deadzone_out] -> Solenoids/4(deadzone_out)
  Solenoids/1(intake) -> [HAM_in]
  Solenoids/2(outtake) -> [HAM_out]
  [k_i] -> PID Controller/3
  [k_d] -> PID Controller/4
  [N] -> PID Controller/5
  Sum/1 -> PID Controller/1
  PID Controller/1 -> Solenoids/1(control)
  [k_p] -> PID Controller/2
  [PAMs_off] -> Solenoids/5(PAMs_on)
  [System_on] -> Solenoids/6(System_on)
  [Depressurize_PAMs] -> Solenoids/7(depressurize)

== system EPA_Jumpe_v1/PAMs/IL ==
  Pressure Des : Inport
  Delay : Delay  DelayLength=1
  PID Controller : simulink/Continuous/PID Controller  Controller=PID  TimeDomain=Discrete-time  SampleTime=-1  IntegratorMethod=Forward Euler  FilterMethod=Forward Euler  Form=Ideal  UseFilter=on  ControllerParametersSource=external  P=k_p_pam  I=0  D=0.45*0.15/8  N=100  InitialConditionSource=internal  InitialConditionForIntegrator=0  InitialConditionForFilter=0  ExternalReset=none  LimitOutput=off  UpperSaturationLimit=inf  LowerSaturationLimit=-inf  LinearizeAsGain=on  AntiWindupMode=none  Kb=1  TrackingMode=off  Kt=1  PParamMin=[]  PParamMax=[]  IParamMin=[]  IParamMax=[]  DParamMin=[]  DParamMax=[]  NParamMin=[]  NParamMax=[]  KbParamMin=[]  KbParamMax=[]  KtParamMin=[]  KtParamMax=[]  POutMin=[]  POutMax=[]  IOutMin=[]  IOutMax=[]  DOutMin=[]  DOutMax=[]  NOutMin=[]  NOutMax=[]  KbOutMin=[]  KbOutMax=[]  KtOutMin=[]  KtOutMax=[]  IntegratorOutMin=[]  IntegratorOutMax=[]  FilterOutMin=[]  FilterOutMax=[]  SumOutMin=[]  SumOutMax=[]  SumI1OutMin=[]  SumI1OutMax=[]  SumI2OutMin=[]  SumI2OutMax=[]  SumI3OutMin=[]  SumI3OutMax=[]  SumDOutMin=[]  SumDOutMax=[]  SaturationOutMin=[]  SaturationOutMax=[]  IntegratorContinuousStateAttributes=''  IntegratorStateMustResolveToSignalObject=off  IntegratorRTWStateStorageClass=Auto  FilterContinuousStateAttributes=''  FilterStateMustResolveToSignalObject=off  FilterRTWStateStorageClass=Auto  DifferentiatorICPrevScaledInput=0  DifferentiatorOutMin=[]  DifferentiatorOutMax=[]  FilterDiffOutCoefMin=[]  FilterDiffOutCoefMax=[]  SumDenOutMin=[]  SumDenOutMax=[]  SumNumOutMin=[]  SumNumOutMax=[]  ReciprocalOutMin=[]  ReciprocalOutMax=[]  DivideOutMin=[]  DivideOutMax=[]  TunerSelectOption=Transfer Function Based (PID Tuner App)
  Solenoids : MATLAB Function  TreatAsAtomicUnit=on
  Sum : Sum  Inputs=|+-
  tag scope: IL_in=global, IL_out=global
  wires:
  Solenoids/3(inside_deadzone_1) -> Delay/1
  Delay/1 -> Solenoids/2(inside_deadzone)
  Pressure Des/1 -> Sum/1
  [IL_pres] -> Sum/2
  [deadzone_in] -> Solenoids/3(deadzone_in)
  [deadzone_out] -> Solenoids/4(deadzone_out)
  Solenoids/1(intake) -> [IL_in]
  Solenoids/2(outtake) -> [IL_out]
  [k_i] -> PID Controller/3
  [k_d] -> PID Controller/4
  [N] -> PID Controller/5
  Sum/1 -> PID Controller/1
  PID Controller/1 -> Solenoids/1(control)
  [k_p] -> PID Controller/2
  [PAMs_off] -> Solenoids/5(PAMs_on)
  [System_on] -> Solenoids/6(System_on)
  [Depressurize_PAMs] -> Solenoids/7(depressurize)

== system EPA_Jumpe_v1/PAMs/POP ==
  Pressure Des : Inport
  Delay : Delay  DelayLength=1
  PID Controller : simulink/Continuous/PID Controller  Controller=PID  TimeDomain=Discrete-time  SampleTime=-1  IntegratorMethod=Forward Euler  FilterMethod=Forward Euler  Form=Ideal  UseFilter=on  ControllerParametersSource=external  P=k_p_pam  I=0  D=0.45*0.15/8  N=100  InitialConditionSource=internal  InitialConditionForIntegrator=0  InitialConditionForFilter=0  ExternalReset=none  LimitOutput=off  UpperSaturationLimit=inf  LowerSaturationLimit=-inf  LinearizeAsGain=on  AntiWindupMode=none  Kb=1  TrackingMode=off  Kt=1  PParamMin=[]  PParamMax=[]  IParamMin=[]  IParamMax=[]  DParamMin=[]  DParamMax=[]  NParamMin=[]  NParamMax=[]  KbParamMin=[]  KbParamMax=[]  KtParamMin=[]  KtParamMax=[]  POutMin=[]  POutMax=[]  IOutMin=[]  IOutMax=[]  DOutMin=[]  DOutMax=[]  NOutMin=[]  NOutMax=[]  KbOutMin=[]  KbOutMax=[]  KtOutMin=[]  KtOutMax=[]  IntegratorOutMin=[]  IntegratorOutMax=[]  FilterOutMin=[]  FilterOutMax=[]  SumOutMin=[]  SumOutMax=[]  SumI1OutMin=[]  SumI1OutMax=[]  SumI2OutMin=[]  SumI2OutMax=[]  SumI3OutMin=[]  SumI3OutMax=[]  SumDOutMin=[]  SumDOutMax=[]  SaturationOutMin=[]  SaturationOutMax=[]  IntegratorContinuousStateAttributes=''  IntegratorStateMustResolveToSignalObject=off  IntegratorRTWStateStorageClass=Auto  FilterContinuousStateAttributes=''  FilterStateMustResolveToSignalObject=off  FilterRTWStateStorageClass=Auto  DifferentiatorICPrevScaledInput=0  DifferentiatorOutMin=[]  DifferentiatorOutMax=[]  FilterDiffOutCoefMin=[]  FilterDiffOutCoefMax=[]  SumDenOutMin=[]  SumDenOutMax=[]  SumNumOutMin=[]  SumNumOutMax=[]  ReciprocalOutMin=[]  ReciprocalOutMax=[]  DivideOutMin=[]  DivideOutMax=[]  TunerSelectOption=Transfer Function Based (PID Tuner App)
  Solenoids : MATLAB Function  TreatAsAtomicUnit=on
  Sum : Sum  Inputs=|+-
  tag scope: POP_in=global, POP_out=global
  wires:
  Solenoids/3(inside_deadzone_1) -> Delay/1
  Delay/1 -> Solenoids/2(inside_deadzone)
  Pressure Des/1 -> Sum/1
  [POP_pres] -> Sum/2
  [deadzone_in_pop] -> Solenoids/3(deadzone_in)
  [deadzone_out_pop] -> Solenoids/4(deadzone_out)
  Solenoids/1(intake) -> [POP_in]
  Solenoids/2(outtake) -> [POP_out]
  [k_i] -> PID Controller/3
  [k_d] -> PID Controller/4
  [N] -> PID Controller/5
  Sum/1 -> PID Controller/1
  PID Controller/1 -> Solenoids/1(control)
  [k_p] -> PID Controller/2
  [PAMs_off] -> Solenoids/5(PAMs_on)
  [System_on] -> Solenoids/6(System_on)
  [Depressurize_PAMs] -> Solenoids/7(depressurize)

== system EPA_Jumpe_v1/PAMs/RF ==
  Pressure Des : Inport
  Delay : Delay  DelayLength=1
  PID Controller : simulink/Continuous/PID Controller  Controller=PID  TimeDomain=Discrete-time  SampleTime=-1  IntegratorMethod=Forward Euler  FilterMethod=Forward Euler  Form=Ideal  UseFilter=on  ControllerParametersSource=external  P=k_p_pam  I=0  D=0.45*0.15/8  N=100  InitialConditionSource=internal  InitialConditionForIntegrator=0  InitialConditionForFilter=0  ExternalReset=none  LimitOutput=off  UpperSaturationLimit=inf  LowerSaturationLimit=-inf  LinearizeAsGain=on  AntiWindupMode=none  Kb=1  TrackingMode=off  Kt=1  PParamMin=[]  PParamMax=[]  IParamMin=[]  IParamMax=[]  DParamMin=[]  DParamMax=[]  NParamMin=[]  NParamMax=[]  KbParamMin=[]  KbParamMax=[]  KtParamMin=[]  KtParamMax=[]  POutMin=[]  POutMax=[]  IOutMin=[]  IOutMax=[]  DOutMin=[]  DOutMax=[]  NOutMin=[]  NOutMax=[]  KbOutMin=[]  KbOutMax=[]  KtOutMin=[]  KtOutMax=[]  IntegratorOutMin=[]  IntegratorOutMax=[]  FilterOutMin=[]  FilterOutMax=[]  SumOutMin=[]  SumOutMax=[]  SumI1OutMin=[]  SumI1OutMax=[]  SumI2OutMin=[]  SumI2OutMax=[]  SumI3OutMin=[]  SumI3OutMax=[]  SumDOutMin=[]  SumDOutMax=[]  SaturationOutMin=[]  SaturationOutMax=[]  IntegratorContinuousStateAttributes=''  IntegratorStateMustResolveToSignalObject=off  IntegratorRTWStateStorageClass=Auto  FilterContinuousStateAttributes=''  FilterStateMustResolveToSignalObject=off  FilterRTWStateStorageClass=Auto  DifferentiatorICPrevScaledInput=0  DifferentiatorOutMin=[]  DifferentiatorOutMax=[]  FilterDiffOutCoefMin=[]  FilterDiffOutCoefMax=[]  SumDenOutMin=[]  SumDenOutMax=[]  SumNumOutMin=[]  SumNumOutMax=[]  ReciprocalOutMin=[]  ReciprocalOutMax=[]  DivideOutMin=[]  DivideOutMax=[]  TunerSelectOption=Transfer Function Based (PID Tuner App)
  Solenoids : MATLAB Function  TreatAsAtomicUnit=on
  Sum : Sum  Inputs=|+-
  tag scope: RF_in=global, RF_out=global
  wires:
  Solenoids/3(inside_deadzone_1) -> Delay/1
  Delay/1 -> Solenoids/2(inside_deadzone)
  Pressure Des/1 -> Sum/1
  [RF_pres] -> Sum/2
  [deadzone_in] -> Solenoids/3(deadzone_in)
  [deadzone_out] -> Solenoids/4(deadzone_out)
  Solenoids/1(intake) -> [RF_in]
  Solenoids/2(outtake) -> [RF_out]
  [k_i] -> PID Controller/3
  [k_d] -> PID Controller/4
  [N] -> PID Controller/5
  Sum/1 -> PID Controller/1
  PID Controller/1 -> Solenoids/1(control)
  [k_p] -> PID Controller/2
  [PAMs_off] -> Solenoids/5(PAMs_on)
  [System_on] -> Solenoids/6(System_on)
  [Depressurize_PAMs] -> Solenoids/7(depressurize)

== system EPA_Jumpe_v1/PAMs/SOL ==
  Pressure Des : Inport
  Delay : Delay  DelayLength=1
  PID Controller : simulink/Continuous/PID Controller  Controller=PID  TimeDomain=Discrete-time  SampleTime=-1  IntegratorMethod=Forward Euler  FilterMethod=Forward Euler  Form=Ideal  UseFilter=on  ControllerParametersSource=external  P=k_p_pam  I=0  D=0.45*0.15/8  N=100  InitialConditionSource=internal  InitialConditionForIntegrator=0  InitialConditionForFilter=0  ExternalReset=none  LimitOutput=off  UpperSaturationLimit=inf  LowerSaturationLimit=-inf  LinearizeAsGain=on  AntiWindupMode=none  Kb=1  TrackingMode=off  Kt=1  PParamMin=[]  PParamMax=[]  IParamMin=[]  IParamMax=[]  DParamMin=[]  DParamMax=[]  NParamMin=[]  NParamMax=[]  KbParamMin=[]  KbParamMax=[]  KtParamMin=[]  KtParamMax=[]  POutMin=[]  POutMax=[]  IOutMin=[]  IOutMax=[]  DOutMin=[]  DOutMax=[]  NOutMin=[]  NOutMax=[]  KbOutMin=[]  KbOutMax=[]  KtOutMin=[]  KtOutMax=[]  IntegratorOutMin=[]  IntegratorOutMax=[]  FilterOutMin=[]  FilterOutMax=[]  SumOutMin=[]  SumOutMax=[]  SumI1OutMin=[]  SumI1OutMax=[]  SumI2OutMin=[]  SumI2OutMax=[]  SumI3OutMin=[]  SumI3OutMax=[]  SumDOutMin=[]  SumDOutMax=[]  SaturationOutMin=[]  SaturationOutMax=[]  IntegratorContinuousStateAttributes=''  IntegratorStateMustResolveToSignalObject=off  IntegratorRTWStateStorageClass=Auto  FilterContinuousStateAttributes=''  FilterStateMustResolveToSignalObject=off  FilterRTWStateStorageClass=Auto  DifferentiatorICPrevScaledInput=0  DifferentiatorOutMin=[]  DifferentiatorOutMax=[]  FilterDiffOutCoefMin=[]  FilterDiffOutCoefMax=[]  SumDenOutMin=[]  SumDenOutMax=[]  SumNumOutMin=[]  SumNumOutMax=[]  ReciprocalOutMin=[]  ReciprocalOutMax=[]  DivideOutMin=[]  DivideOutMax=[]  TunerSelectOption=Transfer Function Based (PID Tuner App)
  Solenoids : MATLAB Function  TreatAsAtomicUnit=on
  Sum : Sum  Inputs=|+-
  tag scope: SOL_in=global, SOL_out=global
  wires:
  Solenoids/3(inside_deadzone_1) -> Delay/1
  Delay/1 -> Solenoids/2(inside_deadzone)
  PID Controller/1 -> Solenoids/1(control)
  Pressure Des/1 -> Sum/1
  [SOL_pres] -> Sum/2
  [deadzone_in] -> Solenoids/3(deadzone_in)
  [deadzone_out] -> Solenoids/4(deadzone_out)
  Solenoids/1(intake) -> [SOL_in]
  Solenoids/2(outtake) -> [SOL_out]
  [k_i] -> PID Controller/3
  [k_d] -> PID Controller/4
  [N] -> PID Controller/5
  Sum/1 -> PID Controller/1
  [k_p] -> PID Controller/2
  [PAMs_off] -> Solenoids/5(PAMs_on)
  [System_on] -> Solenoids/6(System_on)
  [Depressurize_PAMs] -> Solenoids/7(depressurize)

== system EPA_Jumpe_v1/PAMs/TIB ==
  Pressure Des : Inport
  Delay : Delay  DelayLength=1
  PID Controller : simulink/Continuous/PID Controller  Controller=PID  TimeDomain=Discrete-time  SampleTime=-1  IntegratorMethod=Forward Euler  FilterMethod=Forward Euler  Form=Ideal  UseFilter=on  ControllerParametersSource=internal  P=k_p_TIB  I=0  D=0.01  N=300  InitialConditionSource=internal  InitialConditionForIntegrator=0  InitialConditionForFilter=0  ExternalReset=none  LimitOutput=off  UpperSaturationLimit=inf  LowerSaturationLimit=-inf  LinearizeAsGain=on  AntiWindupMode=none  Kb=1  TrackingMode=off  Kt=1  PParamMin=[]  PParamMax=[]  IParamMin=[]  IParamMax=[]  DParamMin=[]  DParamMax=[]  NParamMin=[]  NParamMax=[]  KbParamMin=[]  KbParamMax=[]  KtParamMin=[]  KtParamMax=[]  POutMin=[]  POutMax=[]  IOutMin=[]  IOutMax=[]  DOutMin=[]  DOutMax=[]  NOutMin=[]  NOutMax=[]  KbOutMin=[]  KbOutMax=[]  KtOutMin=[]  KtOutMax=[]  IntegratorOutMin=[]  IntegratorOutMax=[]  FilterOutMin=[]  FilterOutMax=[]  SumOutMin=[]  SumOutMax=[]  SumI1OutMin=[]  SumI1OutMax=[]  SumI2OutMin=[]  SumI2OutMax=[]  SumI3OutMin=[]  SumI3OutMax=[]  SumDOutMin=[]  SumDOutMax=[]  SaturationOutMin=[]  SaturationOutMax=[]  IntegratorContinuousStateAttributes=''  IntegratorStateMustResolveToSignalObject=off  IntegratorRTWStateStorageClass=Auto  FilterContinuousStateAttributes=''  FilterStateMustResolveToSignalObject=off  FilterRTWStateStorageClass=Auto  DifferentiatorICPrevScaledInput=0  DifferentiatorOutMin=[]  DifferentiatorOutMax=[]  FilterDiffOutCoefMin=[]  FilterDiffOutCoefMax=[]  SumDenOutMin=[]  SumDenOutMax=[]  SumNumOutMin=[]  SumNumOutMax=[]  ReciprocalOutMin=[]  ReciprocalOutMax=[]  DivideOutMin=[]  DivideOutMax=[]  TunerSelectOption=Transfer Function Based (PID Tuner App)
  Solenoids : MATLAB Function  TreatAsAtomicUnit=on
  Sum : Sum  Inputs=|+-
  tag scope: TIB_in=global, TIB_out=global
  wires:
  Solenoids/3(inside_deadzone_1) -> Delay/1
  Delay/1 -> Solenoids/2(inside_deadzone)
  Pressure Des/1 -> Sum/1
  [TIB_pres] -> Sum/2
  Solenoids/1(intake) -> [TIB_in]
  Solenoids/2(outtake) -> [TIB_out]
  [PAMs_off] -> Solenoids/3(PAMs_on)
  [System_on] -> Solenoids/4(System_on)
  PID Controller/1 -> Solenoids/1(control)
  Sum/1 -> PID Controller/1
  [Depressurize_PAMs] -> Solenoids/5(depressurize)

== system EPA_Jumpe_v1/PAMs/VAS ==
  Pressure Des : Inport
  Delay : Delay  DelayLength=1
  PID Controller : simulink/Continuous/PID Controller  Controller=PID  TimeDomain=Discrete-time  SampleTime=-1  IntegratorMethod=Forward Euler  FilterMethod=Forward Euler  Form=Ideal  UseFilter=on  ControllerParametersSource=external  P=k_p_pam  I=0  D=0.45*0.15/8  N=100  InitialConditionSource=internal  InitialConditionForIntegrator=0  InitialConditionForFilter=0  ExternalReset=none  LimitOutput=off  UpperSaturationLimit=inf  LowerSaturationLimit=-inf  LinearizeAsGain=on  AntiWindupMode=none  Kb=1  TrackingMode=off  Kt=1  PParamMin=[]  PParamMax=[]  IParamMin=[]  IParamMax=[]  DParamMin=[]  DParamMax=[]  NParamMin=[]  NParamMax=[]  KbParamMin=[]  KbParamMax=[]  KtParamMin=[]  KtParamMax=[]  POutMin=[]  POutMax=[]  IOutMin=[]  IOutMax=[]  DOutMin=[]  DOutMax=[]  NOutMin=[]  NOutMax=[]  KbOutMin=[]  KbOutMax=[]  KtOutMin=[]  KtOutMax=[]  IntegratorOutMin=[]  IntegratorOutMax=[]  FilterOutMin=[]  FilterOutMax=[]  SumOutMin=[]  SumOutMax=[]  SumI1OutMin=[]  SumI1OutMax=[]  SumI2OutMin=[]  SumI2OutMax=[]  SumI3OutMin=[]  SumI3OutMax=[]  SumDOutMin=[]  SumDOutMax=[]  SaturationOutMin=[]  SaturationOutMax=[]  IntegratorContinuousStateAttributes=''  IntegratorStateMustResolveToSignalObject=off  IntegratorRTWStateStorageClass=Auto  FilterContinuousStateAttributes=''  FilterStateMustResolveToSignalObject=off  FilterRTWStateStorageClass=Auto  DifferentiatorICPrevScaledInput=0  DifferentiatorOutMin=[]  DifferentiatorOutMax=[]  FilterDiffOutCoefMin=[]  FilterDiffOutCoefMax=[]  SumDenOutMin=[]  SumDenOutMax=[]  SumNumOutMin=[]  SumNumOutMax=[]  ReciprocalOutMin=[]  ReciprocalOutMax=[]  DivideOutMin=[]  DivideOutMax=[]  TunerSelectOption=Transfer Function Based (PID Tuner App)
  Solenoids : MATLAB Function  TreatAsAtomicUnit=on
  Sum : Sum  Inputs=|+-
  tag scope: VAS_in=global, VAS_out=global
  wires:
  Solenoids/3(inside_deadzone_1) -> Delay/1
  Delay/1 -> Solenoids/2(inside_deadzone)
  Pressure Des/1 -> Sum/1
  [VAS_pres] -> Sum/2
  [deadzone_in] -> Solenoids/3(deadzone_in)
  [deadzone_out] -> Solenoids/4(deadzone_out)
  Solenoids/1(intake) -> [VAS_in]
  [k_i] -> PID Controller/3
  [k_d] -> PID Controller/4
  [N] -> PID Controller/5
  Sum/1 -> PID Controller/1
  PID Controller/1 -> Solenoids/1(control)
  [k_p] -> PID Controller/2
  [PAMs_off] -> Solenoids/5(PAMs_on)
  [System_on] -> Solenoids/6(System_on)
  Solenoids/2(outtake) -> [VAS_out]
  [Depressurize_PAMs] -> Solenoids/7(depressurize)

== system EPA_Jumpe_v1/Safety /System On ==
  "Simulink Switch " : Inport
  Clock2 : Clock
  Compare To Constant : simulink/Logic and Bit Operations/Compare To Constant  relop=>=  const=10  OutDataTypeStr=boolean
  Data Type Conversion3 : DataTypeConversion  OutDataTypeStr=double
  Emergency Switch : MATLAB Function  TreatAsAtomicUnit=on
  Logical Operator : Logic  Inputs=3  AllPortsSameDT=off  OutDataTypeStr=boolean
  System On : Outport
  Emergency : Outport  Port=2
  wires:
  Emergency Switch/1(y) -> Emergency/1, Logical Operator/3
  [Emergency_Switch] -> Emergency Switch/1(Emergency_switch)
  "Simulink Switch "/1 -> Logical Operator/2
  Clock2/1 -> Compare To Constant/1
  Compare To Constant/1 -> Logical Operator/1
  Logical Operator/1 -> Data Type Conversion3/1
  Data Type Conversion3/1 -> System On/1

== system EPA_Jumpe_v1/Ethernet Communication/Inputs/GRF Slave ==
  note: Emergency Switch
  note: GRF
  Data Type Conversion3 : DataTypeConversion
  EtherCAT PDO Receive1 : xpcethercatlib/EtherCAT PDO Receive  Priority=2  sig_name=GRF.Inputs.Byte13  sig_offset=312  sig_type=uint8  type_size=8  sig_dim=1  device_id=0  sample_time=0.001000
      settings: SourceProductName=Simulink Real-Time  SourceProductBaseCode=XP
  EtherCAT PDO Receive2 : xpcethercatlib/EtherCAT PDO Receive  Priority=2  sig_name=GRF.Inputs.Byte14  sig_offset=320  sig_type=uint8  type_size=8  sig_dim=1  device_id=0  sample_time=0.001000
      settings: SourceProductName=Simulink Real-Time  SourceProductBaseCode=XP
  "GRFx " : Subsystem
  "GRFy " : Subsystem
  "GRFz " : Subsystem
  Gain24 : Gain  Gain=256
  Sum5 : Sum
  tag scope: Emergency_Switch=global
  wires:
  Data Type Conversion3/1 -> [Emergency_Switch]
  Gain24/1 -> Sum5/1
  EtherCAT PDO Receive2/1 -> Sum5/2
  Sum5/1 -> Data Type Conversion3/1
  EtherCAT PDO Receive1/1 -> Gain24/1
